simulink library "Mylibrary"  (R2019b)
settings: Solver=VariableStepAuto  StartTime=0.0  StopTime=10.0  RelTol=1e-3
settings Model: Creator=hezhaoyang  LastModifiedBy=86156

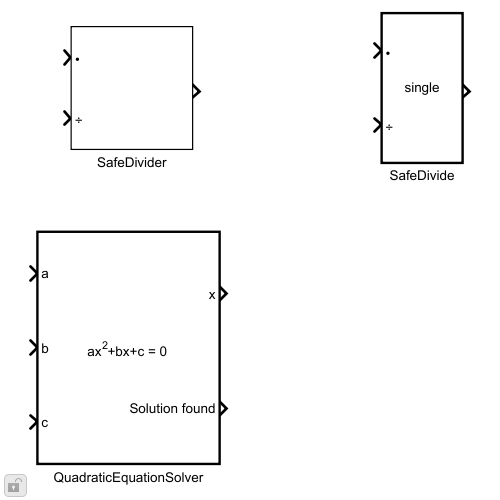
[thumbnail: Simulink's stored preview of the top-level diagram]
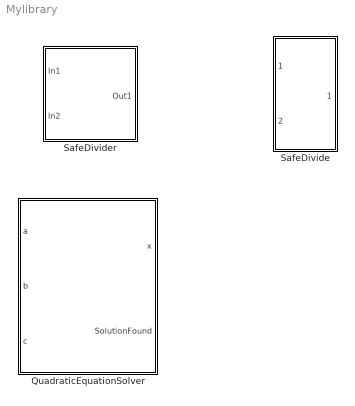
== system Mylibrary ==
  QuadraticEquationSolver : MATLAB Function  TreatAsAtomicUnit=on  RTWFileName=QuadraticEquationSolverNew  mask(Quadratic equation solver){ZeroThreshold=single(1e-2)}
      mask prompts: ZeroThreshold "Zero threshold:"
      mask help:
      | This block solves a quadratic polynomial equation.
      | Both solutions are returned in a bus.
      | If the equation lacks real roots then zeros are returned,
      | along with a flag indicating that no solutions where found.
      settings: RTWFcnNameOpts=Use subsystem name
  SafeDivide : Subsystem  TreatAsAtomicUnit=on  mask(Safe divide){DataType=single, DataTypeMax=0, DataTypeMin=0}
      mask prompts: DataType "Data type:"
      mask help:
      | This block offers division protected from division by zero.
      |
      | When division by zero is detected, a very large number will be returned with the same sign as the numerator.
      |
      | In the case zero divided by zero, the output has been defined as zero.
      |
      | Both floating-point numbers and integers are supported.
      mask init:
      | % Author: Jakob Andersson (jande573)
      | 
      | % Test if the selected data type is a floating point type or an integer
      | % The supported data types is selected on the parameters pane
      | if(strcmp(DataType,'double')||strcmp(DataType,'single'))
      |     % Find the max and min values of the selected data type
      |     DataTypeMax=fix(sqrt(realmax(DataType))); % In order to avoid errors when operating on the output
      |     DataTypeMin=-fix(sqrt(realmax(DataType))); % In order to avoid errors when operating on the output
      | else
      |     % Find the max and min values of the selected data type
      |     DataTypeMax=intmax(DataType);
      |     DataTypeMin=-intmax(DataType);
      | end
      settings: RTWSystemCode=Inline
      mask Help:
      | This block offers division protected from division by zero.
      | 
      | When division by zero is detected, a very large number will be returned with the same sign as the numerator.
      | 
      | In the case zero divided by zero, the output has been defined as zero.
      | 
      | Both floating-point numbers and integers are supported.
      mask Display:
      | % Author: Jakob Andersson (jande573)
      | 
      | % Display the allowed data type
      | disp(DataType);
      | 
      | % Display the port symbols
      | port_label('input',1,'\bullet','texmode','on');
      | port_label('input',2,'\div','texmode','on');
  SafeDivider : Subsystem
      mask Display:
      | % Display the port symbols
      | port_label('input',1,'\bullet','texmode','on');
      | port_label('input',2,'\div','texmode','on');

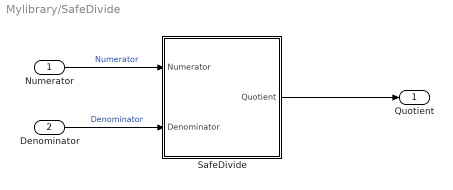
== system Mylibrary/SafeDivide ==
  Numerator : Inport  OutDataTypeStr=DataType
      settings: AttributesFormatString=DT=%<OutDataTypeStr>
  Denominator : Inport  Port=2  OutDataTypeStr=DataType
      settings: AttributesFormatString=DT=%<OutDataTypeStr>
  SafeDivide : MATLAB Function
  Quotient : Outport  OutDataTypeStr=DataType
      settings: AttributesFormatString=DT=%<OutDataTypeStr>
  wires:
  SafeDivide/1(Quotient) -> Quotient/1
  Denominator/1 -> SafeDivide/2(Denominator)  "Denominator"
  Numerator/1 -> SafeDivide/1(Numerator)  "Numerator"

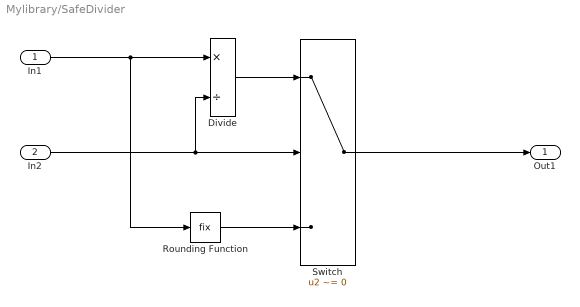
== system Mylibrary/SafeDivider ==
  In1 : Inport
  In2 : Inport  Port=2
  Divide : Product  Inputs=*/
  Rounding Function : Rounding  Operator=fix
  Switch : Switch  Criteria=u2 ~= 0
  Out1 : Outport
  wires:
  In1/1 -> Rounding Function/1, Divide/1
  In2/1 -> Divide/2, Switch/2
  Rounding Function/1 -> Switch/3
  Switch/1 -> Out1/1
  Divide/1 -> Switch/1

== matlab function Mylibrary/QuadraticEquationSolver ==
  data: a input single; x output single; b input single; c input single; SolutionFound output boolean; ZeroThreshold parameter single
function [x, SolutionFound] = fcn(a, b, c, ZeroThreshold)
%#codegen

% Solve ax^2 + bx + c = 0.
% Output x = [x1, x2], where x1 >= x2.

% Case a == 0 and b == 0: Solve c = 0.
aEqualsZero = equalsZero(a, ZeroThreshold);
if aEqualsZero && equalsZero(b, ZeroThreshold)
    
    % Only possible solution exists when also c == 0.
    SolutionFound = equalsZero(c, ZeroThreshold);
    x = single([0; 0]);

% Case a == 0: Solve bx + c = 0.
elseif aEqualsZero
    
    SolutionFound = true;
    x = [-c/b; -c/b];

% Solve the quadratic equation.
% x = (-b ± sqrt(b^2 - 4ac))/(2a).
else
    
    % Complex solutions are not valid.
    bSquared = b*b;
    if 4*a*c > bSquared
        SolutionFound = false;
        x = single([0; 0]);
    else
        SolutionFound = true;
        squareRoot = single(sqrt(bSquared - 4*a*c));
        x1 = (-b + squareRoot)/(2*a); 
        x2 = (-b - squareRoot)/(2*a);
        if x1 > x2
            x = [x1; x2];
        else
            x = [x2; x1];
        end
    end    
end
    
end

% Subfunction equalsZero

function tf = equalsZero(c, ZeroThreshold)

tf = (c < ZeroThreshold && c > -ZeroThreshold);

end

== matlab function Mylibrary/SafeDivide/SafeDivide ==
  data: Numerator input; Quotient output; Denominator input; DataTypeMin parameter; DataTypeMax parameter
function Quotient = fcn(Numerator, Denominator, DataTypeMin, DataTypeMax)
    %#codegen
    
    % Test for division by zero and overflow
    if abs(Denominator) > abs(Numerator)*(1/DataTypeMax)
        % Normal divide
        Quotient=Numerator/Denominator;
    else
        % Select output depending on the numerator
        if Numerator>0
            % x/0
            Quotient=DataTypeMax;
        elseif Numerator<0
            % -x/0
            Quotient=DataTypeMin;
        else
            % 0/0
            Quotient=cast(0,class(Numerator));
        end
    end
end
